simulink model "Wheel3D"  (R2022a)
settings: Solver=VariableStepAuto  StartTime=0.0  StopTime=15  RelTol=1e-3
undefined symbols (not defined in the file): DiscIntNeverNeededParam
libraries: simulink_extras x2, aerolibanimutils x1, vrlib x1
settings Model: ExtModeTrigDuration=5001  Creator=l.alloza  LastModifiedBy=fades
settings SolverCC: AlgebraicLoopSolver=TrustRegion
settings DataIOCC: SaveFormat=Array  SaveOutput=off  SignalLogging=off  DSMLogging=off  SaveTime=off  ReturnWorkspaceOutputs=off
settings DebuggingCC: UnderspecifiedInitializationDetection=Classic  MergeDetectMultiDrivingBlocksExec=none  UnconnectedInputMsg=warning  UnconnectedOutputMsg=warning  UnconnectedLineMsg=warning  SFMachineParentedDataDiag=warning  ArithmeticOperatorsInVariantConditions=warning
settings ModelReferenceCC: PropagateSignalLabelsOutOfModel=off
settings SFSimCC: SimUseLocalCustomCode=off  CustomCodeUndefinedFunction=UseInterfaceOnly
settings RTWCC: RTWUseLocalCustomCode=off

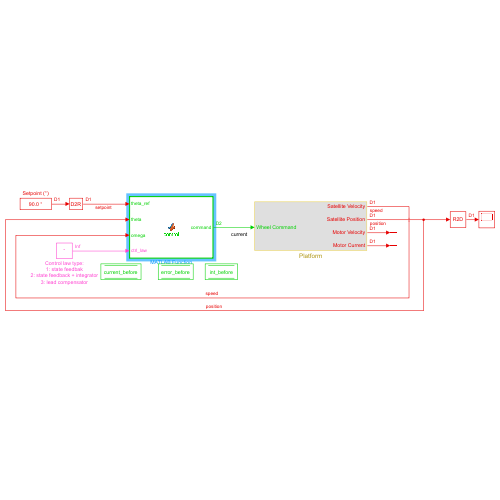
[thumbnail: Simulink's stored preview of the top-level diagram]
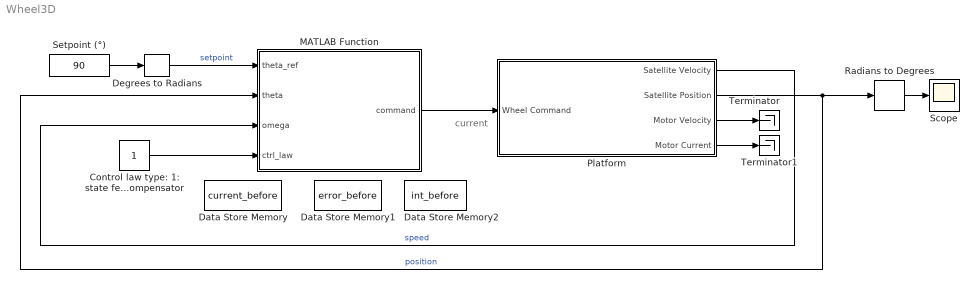
== system Wheel3D ==
  note: current
  Control law type: 1: state feedbak 2: state feedback + integrator 3: lead compensator : Constant  SampleTime=Inf
  Data Store Memory : DataStoreMemory  DataStoreName=current_before  ReadBeforeWriteMsg=warning  WriteAfterWriteMsg=warning  WriteAfterReadMsg=warning  ShowAdditionalParam=off  OutDataTypeStr=double
  Data Store Memory1 : DataStoreMemory  DataStoreName=error_before  ReadBeforeWriteMsg=warning  WriteAfterWriteMsg=warning  WriteAfterReadMsg=warning  ShowAdditionalParam=off  OutDataTypeStr=double
  Data Store Memory2 : DataStoreMemory  DataStoreName=int_before  ReadBeforeWriteMsg=warning  WriteAfterWriteMsg=warning  WriteAfterReadMsg=warning  ShowAdditionalParam=off  OutDataTypeStr=double
  Degrees to Radians : simulink_extras/Transformations/Degrees to Radians
  MATLAB Function : MATLAB Function  TreatAsAtomicUnit=on  SystemSampleTime=0.1
  Platform : Subsystem
  Radians to Degrees : simulink_extras/Transformations/Radians to Degrees
  Scope : Scope
  Setpoint (°) : Constant  Value=90  SampleTime=0.01
      mask Display: fprintf('%.1f °',str2num(get_param(gcb,'Value')));
  Terminator : Terminator
  Terminator1 : Terminator
  wires:
  Platform/2(Satellite Position) -> Radians to Degrees/1, MATLAB Function/2(theta)  "position"
  Platform/1(Satellite Velocity) -> MATLAB Function/3(omega)  "speed"
  Setpoint (°)/1 -> Degrees to Radians/1
  Degrees to Radians/1 -> MATLAB Function/1(theta_ref)  "setpoint"
  Platform/3(Motor Velocity) -> Terminator/1
  Platform/4(Motor Current) -> Terminator1/1
  Control law type: 1: state feedbak 2: state feedback + integrator 3: lead compensator/1 -> MATLAB Function/4(ctrl_law)
  Radians to Degrees/1 -> Scope/1
  MATLAB Function/1(command) -> Platform/1(Wheel Command)

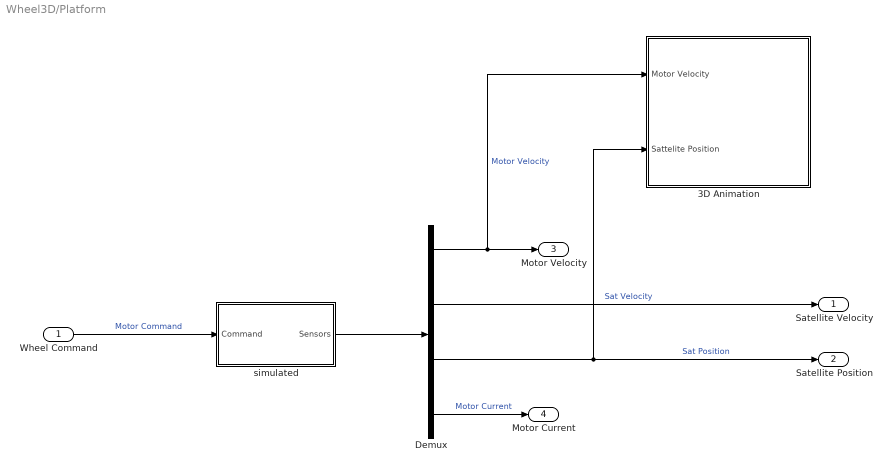
== system Wheel3D/Platform ==
  Wheel Command : Inport
  3D Animation : Subsystem
  Demux : Demux
  simulated : Subsystem  VariantControl=SIMULATED
  Satellite Velocity : Outport  VectorParamsAs1DForOutWhenUnconnected=off
  Satellite Position : Outport  Port=2  VectorParamsAs1DForOutWhenUnconnected=off
  Motor Velocity : Outport  Port=3  VectorParamsAs1DForOutWhenUnconnected=off
  Motor Current : Outport  Port=4  VectorParamsAs1DForOutWhenUnconnected=off
  wires:
  Demux/3 -> 3D Animation/2(Sattelite Position), Satellite Position/1  "Sat Position"
  Demux/2 -> Satellite Velocity/1  "Sat Velocity"
  Demux/4 -> Motor Current/1  "Motor Current"
  Demux/1 -> 3D Animation/1(Motor Velocity), Motor Velocity/1  "Motor Velocity"
  Wheel Command/1 -> simulated/1(Command)  "Motor Command"
  simulated/1(Sensors) -> Demux/1

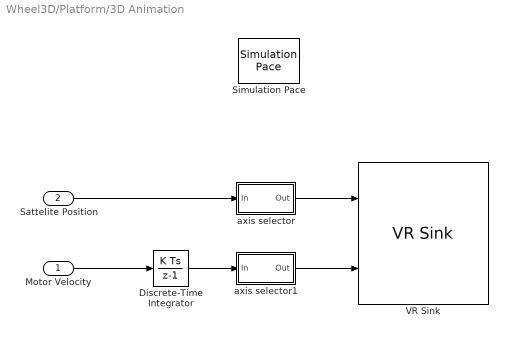
== system Wheel3D/Platform/3D Animation ==
  Motor Velocity : Inport
  Sattelite Position : Inport  Port=2
  Discrete-Time Integrator : DiscreteIntegrator  SampleTime=-1  ICPrevOutput=DiscIntNeverNeededParam  ICPrevScaledInput=DiscIntNeverNeededParam
  Simulation Pace : aerolibanimutils/Simulation Pace  SimulationPace=1  SleepMode=MATLAB Thread  OutputPaceError=off  SampleTime=0.01
  VR Sink : vrlib/VR Sink  InstantiateOnLoad=on  SampleTime=-1  ViewEnable=on  RemoteChange=off  RemoteView=off  FieldsWritten=Platform.rotation.4.1.1.double#Roue.rotation.4.1.1.double  WorldFileName=wheel.wrl  AutoView=on  VideoDimensions=[]  AllowVariableSize=off  FigureProperties="{'Position', 'Name', 'Viewpoint', 'CameraBound', 'CameraDirection', 'CameraPosition', 'CameraUpVector', 'ZoomFactor', 'Antialiasing', 'Headlight', 'Lighting', 'NavPanel', 'Sound', 'StatusBar', 'Stereo3D', 'Stereo3DCameraOffset', 'Stereo3DHIT', 'ToolBar', 'Textures', 'Transparency', 'Triad', 'Wireframe', 'NavZones', 'NavMode', 'NavSpeed', 'CaptureFileFormat', 'CaptureFileName', 'Record2DCompressMethod', 'Record2DCompressQuality', 'Record2D', 'Record2DFileName', 'Record2DFPS'; [2.0000000000000000e+00   8.4000000000000000e+01   9.5800000000000000e+02   8.9600000000000000e+02], 'Reaction Wheel', 'Perspective', 'on', [0.0000000000000000e+00   0.0000000000000000e+00  -1.0000000000000000e+00], [0.0000000000000000e+00   0.0000000000000000e+00   0.0000000000000000e+00], [0.0000000000000000e+00   1.0000000000000000e+00   0.0000000000000000e+00], [1.0000000000000000e+00], 'on', 'on', 'on', 'halfbar', 'on', 'on', 'off', [1.0000000149011612e-01], [0.0000000000000000e+00], 'on', 'on', 'on', 'none', 'off', 'off', 'fly', 'normal', 'tif', '%f_anim_%n.tif', 'auto', [7.5000000000000000e+01], 'off', '%f_anim_%n.avi', 'auto'}"
  axis selector : Subsystem  mask{axdir=Y}
      mask prompts: axdir "Select Direction for output"
      mask init:
      | switch axdir
      |     case 1
      |         v3d = [1 0 0];
      |     case 2
      |         v3d = [0 1 0];
      |     case 3
      |         v3d = [0 0 1];
      | end
      mask TypeOptions axdir: X | Y | Z
      mask Display: disp(get_param(gcb,'axdir'));
  axis selector1 : Subsystem  mask{axdir=Y}
      mask prompts: axdir "Select Direction for output"
      mask init:
      | switch axdir
      |     case 1
      |         v3d = [1 0 0];
      |     case 2
      |         v3d = [0 1 0];
      |     case 3
      |         v3d = [0 0 1];
      | end
      mask TypeOptions axdir: X | Y | Z
      mask Display: disp(get_param(gcb,'axdir'));
  wires:
  Sattelite Position/1 -> axis selector/1(In)
  axis selector1/1(Out) -> VR Sink/2
  axis selector/1(Out) -> VR Sink/1
  Discrete-Time Integrator/1 -> axis selector1/1(In)
  Motor Velocity/1 -> Discrete-Time Integrator/1

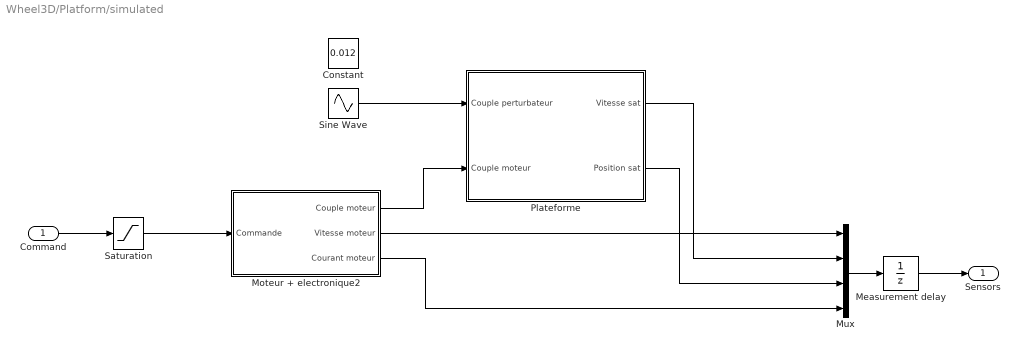
== system Wheel3D/Platform/simulated ==
  Command : Inport
  Constant : Constant  Value=0.012
  Measurement delay : UnitDelay  SampleTime=0.01  HasFrameUpgradeWarning=on
  Moteur + electronique2 : Subsystem
  Mux : Mux
  Plateforme : Subsystem
  Saturation : Saturate  UpperLimit=0.6  LowerLimit=-0.6
  Sine Wave : Sin  Amplitude=0.012  Frequency=0.01  SampleTime=0
  Sensors : Outport  VectorParamsAs1DForOutWhenUnconnected=off
  wires:
  Moteur + electronique2/2(Vitesse moteur) -> Mux/1
  Moteur + electronique2/1(Couple moteur) -> Plateforme/2(Couple moteur)
  Plateforme/1(Vitesse sat) -> Mux/2
  Command/1 -> Saturation/1
  Plateforme/2(Position sat) -> Mux/3
  Saturation/1 -> Moteur + electronique2/1(Commande)
  Moteur + electronique2/3(Courant moteur) -> Mux/4
  Mux/1 -> Measurement delay/1
  Measurement delay/1 -> Sensors/1
  Sine Wave/1 -> Plateforme/1(Couple perturbateur)

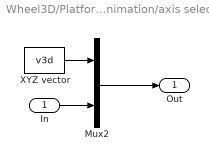
== system Wheel3D/Platform/3D Animation/axis selector ==
  In : Inport
  Mux2 : Mux  Inputs=2
  XYZ vector : Constant  Value=v3d
  Out : Outport  VectorParamsAs1DForOutWhenUnconnected=off
  wires:
  Mux2/1 -> Out/1
  In/1 -> Mux2/2
  XYZ vector/1 -> Mux2/1

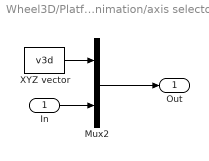
== system Wheel3D/Platform/3D Animation/axis selector1 ==
  In : Inport
  Mux2 : Mux  Inputs=2
  XYZ vector : Constant  Value=v3d
  Out : Outport  VectorParamsAs1DForOutWhenUnconnected=off
  wires:
  XYZ vector/1 -> Mux2/1
  In/1 -> Mux2/2
  Mux2/1 -> Out/1

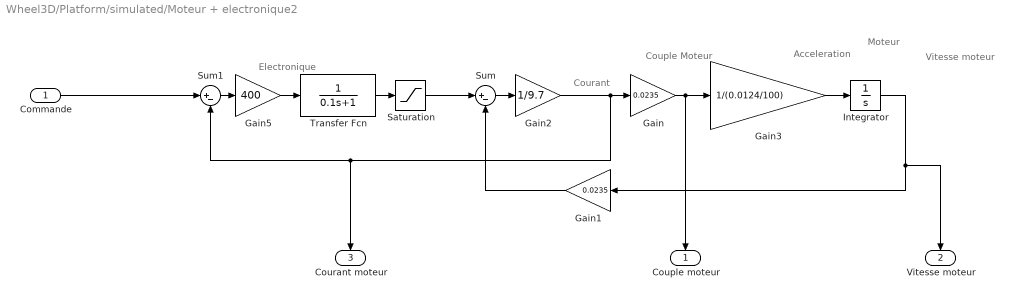
== system Wheel3D/Platform/simulated/Moteur + electronique2 ==
  note: Courant
  note: Couple Moteur
  note: Acceleration
  note: Vitesse
      | moteur
  note: Electronique
  note: Moteur
  Commande : Inport
  Gain : Gain  Gain=0.0235
  Gain1 : Gain  Gain=0.0235
  Gain2 : Gain  Gain=1/9.7
  Gain3 : Gain  Gain=1/(0.0124/100)
  Gain5 : Gain  Gain=400
  Integrator : Integrator
  Saturation : Saturate  UpperLimit=12  LowerLimit=-12
  Sum : Sum  Inputs=|+-
  Sum1 : Sum  Inputs=|+-
  Transfer Fcn : TransferFcn  Denominator=[0.1 1]
  Couple moteur : Outport  VectorParamsAs1DForOutWhenUnconnected=off
  Vitesse moteur : Outport  Port=2  VectorParamsAs1DForOutWhenUnconnected=off
  Courant moteur : Outport  Port=3  VectorParamsAs1DForOutWhenUnconnected=off
  wires:
  Gain3/1 -> Integrator/1
  Gain/1 -> Gain3/1, Couple moteur/1
  Gain2/1 -> Gain/1, Courant moteur/1, Sum1/2
  Sum/1 -> Gain2/1
  Gain1/1 -> Sum/2
  Integrator/1 -> Gain1/1, Vitesse moteur/1
  Gain5/1 -> Transfer Fcn/1
  Sum1/1 -> Gain5/1
  Transfer Fcn/1 -> Saturation/1
  Saturation/1 -> Sum/1
  Commande/1 -> Sum1/1

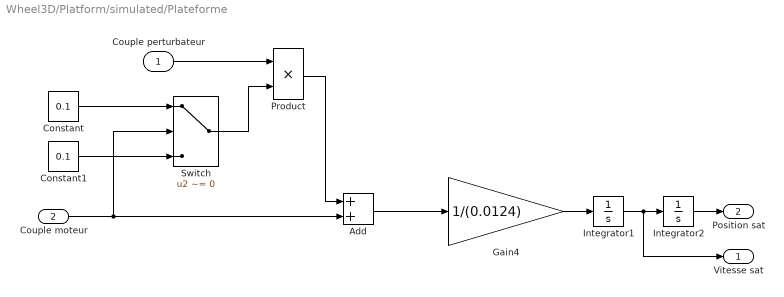
== system Wheel3D/Platform/simulated/Plateforme ==
  Couple perturbateur : Inport
  Couple moteur : Inport  Port=2
  Add : Sum
  Constant : Constant  Value=0.1
  Constant1 : Constant  Value=0.1
  Gain4 : Gain  Gain=1/(0.0124)
  Integrator1 : Integrator
  Integrator2 : Integrator
  Product : Product  RndMeth=Zero
  Switch : Switch  Criteria=u2 ~= 0  SaturateOnIntegerOverflow=off  InputSameDT=off
  Vitesse sat : Outport  VectorParamsAs1DForOutWhenUnconnected=off
  Position sat : Outport  Port=2  VectorParamsAs1DForOutWhenUnconnected=off
  wires:
  Gain4/1 -> Integrator1/1
  Integrator1/1 -> Vitesse sat/1, Integrator2/1
  Integrator2/1 -> Position sat/1
  Add/1 -> Gain4/1
  Couple moteur/1 -> Switch/2, Add/2
  Product/1 -> Add/1
  Couple perturbateur/1 -> Product/1
  Switch/1 -> Product/2
  Constant/1 -> Switch/1
  Constant1/1 -> Switch/3

== matlab function Wheel3D/MATLAB Function ==
  data: theta_ref input; command output; theta input; omega input; ctrl_law input; current_before data_store_memory; error_before data_store_memory; int_before data_store_memory
function command = control(theta_ref, theta, omega, ctrl_law)

% global variables to memorize previous values
global current_before
global error_before
global int_before
current = 0;

%% DEFINE YOUR GAIN VALUES HERE
% state feedback
Kp = 13.1915;
Kv = 4.7489;

% state feedback + integrator
Kii = -3.8466; % integral gain
Kpi = 6.4111;
Kvi = 3.0921;
Te = 0.05; % activation period

% lead compensator
A = 4.291;
B = -4.12;
C = -0.8289;

%% DEFINE YOUR DISCRETE CONTROL LAWS HERE
% statefeedback
if ctrl_law == 1
    current = Kp*(theta_ref - theta) - Kv*omega;
end

% statefeedback + discrete integrator
if ctrl_law == 2
    error = theta_ref - theta;
    int = (Te/2)*(error + error_before) + int_before
    current = -Kii*int - Kpi*theta - Kvi*omega;
    int_before = int;
    error_before = error;
end

% discrete lead compensation
if ctrl_law == 3
    error = theta_ref - theta;
    current = A*error + B*error_before - C*current_before;
    current_before = current;
    error_before = error;
end

%% OUTPUT 
command = current;
